simulink model "idq"  (R2021a)
settings: Solver=VariableStepAuto  StartTime=0.0  StopTime=0.2  FixedStep=1/150000  MaxStep=1e-6
undefined symbols (not defined in the file): in, ou
libraries: neural x105, spsMosfetLib x12, simulink x5, pid_lib x3, spsabctodq0Lib x3, spsFirstOrderFilterLib x2, spsPermanentMagnetSynchronousMachineLib x2, spsCurrentMeasurementLib x2, spsDCVoltageSourceLib x2, spsThreePhaseVIMeasurementLib x2, spsabctoAlphaBetaZeroLib x2, spsSVPWMGenerator2LevelLib x1
(part 5 of 7)

== system idq/NARX Neural Network - Closed Loop1/Layer 2/Delays 1 ==
  "p{2}" : Inport  PortDimensions=10  SampleTime=1e-05
      mask Display: e = 0.06;c1 = [120 230 180]/255;c2 = ([120 230 180]+0)/(256+128);c3 = ([120 230 180]+128)/(256+128);patch([0 1 1 0],[0 0 1 1],c1);patch([0 1 1 1-e 1-e 0+e],[0 0 1 1-e 0+e 0+e],c2);patch([0 0 1 1-e 0+e 0+e],[0 1 1 1-e 1-e 0+e],c3);plot([0 1 1 0 0],[0 0 1 1 0]);
  mux : Mux  Inputs=1
      mask Display: e = 0.06;c1 = [120 150 230]/255;c2 = ([120 150 230]+0)/383;c3 = ([120 150 230]+128)/383;patch([0 1 1 0],[0 0 1 1],c1);patch([0 1 1 1-e 1-e 0+e],[0 0 1 1-e 0+e 0+e],c2);patch([0 0 1 1-e 0+e 0+e],[0 1 1 1-e 1-e 0+e],c3);plot([0 1 1 0 0],[0 0 1 1 0]);disp('Mux')
  "pd{2,1}" : Outport
      mask Display: e = 0.06;c1 = [120 230 180]/255;c2 = ([120 230 180]+0)/(256+128);c3 = ([120 230 180]+128)/(256+128);patch([0 1 1 0],[0 0 1 1],c1);patch([0 1 1 1-e 1-e 0+e],[0 0 1 1-e 0+e 0+e],c2);patch([0 0 1 1-e 0+e 0+e],[0 1 1 1-e 1-e 0+e],c3);plot([0 1 1 0 0],[0 0 1 1 0]);
  wires:
  "p{2}"/1 -> mux/1
  mux/1 -> "pd{2,1}"/1

== system idq/NARX Neural Network - Closed Loop1/Layer 2/LW{2,1} ==
  "ad{2,1}" : Inport  PortDimensions=10  SampleTime=1e-05
      mask Display: e = 0.06;c1 = [120 230 180]/255;c2 = ([120 230 180]+0)/(256+128);c3 = ([120 230 180]+128)/(256+128);patch([0 1 1 0],[0 0 1 1],c1);patch([0 1 1 1-e 1-e 0+e],[0 0 1 1-e 0+e 0+e],c2);patch([0 0 1 1-e 0+e 0+e],[0 1 1 1-e 1-e 0+e],c3);plot([0 1 1 0 0],[0 0 1 1 0]);
  "IW{2,1}(1,:)'" : Constant  Value=[0.56153761305586458174587960456847213208675384521484375;0.83032986406449749150482375625870190560817718505859375;1.7572116988873085485778346992447040975093841552734375;-1.22353547781027049978774812188930809497833251953125;0.69692667626243232081861833648872561752796173095703125;1.5315847736811942780832396238110959529876708984375;-1.373036182446984110328003225731663405895233154296875;1.3479512008090404062699008136405609548091888427734375;1.708104159078249306702446119743399322032928466796875;-0.5444366534227558229730448147165589034557342529296875]
      mask Display: e = 0.06;c1 = [120 150 230]/255;c2 = ([120 150 230]+0)/383;c3 = ([120 150 230]+128)/383;patch([0 1 1 0],[0 0 1 1],c1);patch([0 1 1 1-e 1-e 0+e],[0 0 1 1-e 0+e 0+e],c2);patch([0 0 1 1-e 0+e 0+e],[0 1 1 1-e 1-e 0+e],c3);plot([0 1 1 0 0],[0 0 1 1 0]);disp('weights');
  Mux : Mux  Inputs=1
      mask Display: e = 0.06;c1 = [120 150 230]/255;c2 = ([120 150 230]+0)/383;c3 = ([120 150 230]+128)/383;patch([0 1 1 0],[0 0 1 1],c1);patch([0 1 1 1-e 1-e 0+e],[0 0 1 1-e 0+e 0+e],c2);patch([0 0 1 1-e 0+e 0+e],[0 1 1 1-e 1-e 0+e],c3);plot([0 1 1 0 0],[0 0 1 1 0]);disp('Mux');
  dotprod1 : neural/Weight Functions/dotprod
  "lz{2,1}" : Outport
      mask Display: e = 0.06;c1 = [120 230 180]/255;c2 = ([120 230 180]+0)/(256+128);c3 = ([120 230 180]+128)/(256+128);patch([0 1 1 0],[0 0 1 1],c1);patch([0 1 1 1-e 1-e 0+e],[0 0 1 1-e 0+e 0+e],c2);patch([0 0 1 1-e 0+e 0+e],[0 1 1 1-e 1-e 0+e],c3);plot([0 1 1 0 0],[0 0 1 1 0]);
  wires:
  "IW{2,1}(1,:)'"/1 -> dotprod1/1
  "ad{2,1}"/1 -> dotprod1/2
  dotprod1/1 -> Mux/1
  Mux/1 -> "lz{2,1}"/1

== system idq/NARX Neural Network - Closed Loop2/Layer 1/Delays 1 ==
  "p{1}" : Inport  PortDimensions=4  SampleTime=1e-05
      mask Display: e = 0.06;c1 = [120 230 180]/255;c2 = ([120 230 180]+0)/(256+128);c3 = ([120 230 180]+128)/(256+128);patch([0 1 1 0],[0 0 1 1],c1);patch([0 1 1 1-e 1-e 0+e],[0 0 1 1-e 0+e 0+e],c2);patch([0 0 1 1-e 0+e 0+e],[0 1 1 1-e 1-e 0+e],c3);plot([0 1 1 0 0],[0 0 1 1 0]);
  Delay 1 : UnitDelay  InitialCondition=pi_input_1_delayed_1  SampleTime=1e-05
      mask Display: e = 0.06;c1 = [120 150 230]/255;c2 = ([120 150 230]+0)/383;c3 = ([120 150 230]+128)/383;patch([0 1 1 0],[0 0 1 1],c1);patch([0 1 1 1-e 1-e 0+e],[0 0 1 1-e 0+e 0+e],c2);patch([0 0 1 1-e 0+e 0+e],[0 1 1 1-e 1-e 0+e],c3);plot([0 1 1 0 0],[0 0 1 1 0]);disp('D')
  Delay 10 : UnitDelay  InitialCondition=pi_input_1_delayed_10  SampleTime=1e-05
      mask Display: e = 0.06;c1 = [120 150 230]/255;c2 = ([120 150 230]+0)/383;c3 = ([120 150 230]+128)/383;patch([0 1 1 0],[0 0 1 1],c1);patch([0 1 1 1-e 1-e 0+e],[0 0 1 1-e 0+e 0+e],c2);patch([0 0 1 1-e 0+e 0+e],[0 1 1 1-e 1-e 0+e],c3);plot([0 1 1 0 0],[0 0 1 1 0]);disp('D')
  Delay 2 : UnitDelay  InitialCondition=pi_input_1_delayed_2  SampleTime=1e-05
      mask Display: e = 0.06;c1 = [120 150 230]/255;c2 = ([120 150 230]+0)/383;c3 = ([120 150 230]+128)/383;patch([0 1 1 0],[0 0 1 1],c1);patch([0 1 1 1-e 1-e 0+e],[0 0 1 1-e 0+e 0+e],c2);patch([0 0 1 1-e 0+e 0+e],[0 1 1 1-e 1-e 0+e],c3);plot([0 1 1 0 0],[0 0 1 1 0]);disp('D')
  Delay 3 : UnitDelay  InitialCondition=pi_input_1_delayed_3  SampleTime=1e-05
      mask Display: e = 0.06;c1 = [120 150 230]/255;c2 = ([120 150 230]+0)/383;c3 = ([120 150 230]+128)/383;patch([0 1 1 0],[0 0 1 1],c1);patch([0 1 1 1-e 1-e 0+e],[0 0 1 1-e 0+e 0+e],c2);patch([0 0 1 1-e 0+e 0+e],[0 1 1 1-e 1-e 0+e],c3);plot([0 1 1 0 0],[0 0 1 1 0]);disp('D')
  Delay 4 : UnitDelay  InitialCondition=pi_input_1_delayed_4  SampleTime=1e-05
      mask Display: e = 0.06;c1 = [120 150 230]/255;c2 = ([120 150 230]+0)/383;c3 = ([120 150 230]+128)/383;patch([0 1 1 0],[0 0 1 1],c1);patch([0 1 1 1-e 1-e 0+e],[0 0 1 1-e 0+e 0+e],c2);patch([0 0 1 1-e 0+e 0+e],[0 1 1 1-e 1-e 0+e],c3);plot([0 1 1 0 0],[0 0 1 1 0]);disp('D')
  Delay 5 : UnitDelay  InitialCondition=pi_input_1_delayed_5  SampleTime=1e-05
      mask Display: e = 0.06;c1 = [120 150 230]/255;c2 = ([120 150 230]+0)/383;c3 = ([120 150 230]+128)/383;patch([0 1 1 0],[0 0 1 1],c1);patch([0 1 1 1-e 1-e 0+e],[0 0 1 1-e 0+e 0+e],c2);patch([0 0 1 1-e 0+e 0+e],[0 1 1 1-e 1-e 0+e],c3);plot([0 1 1 0 0],[0 0 1 1 0]);disp('D')
  Delay 6 : UnitDelay  InitialCondition=pi_input_1_delayed_6  SampleTime=1e-05
      mask Display: e = 0.06;c1 = [120 150 230]/255;c2 = ([120 150 230]+0)/383;c3 = ([120 150 230]+128)/383;patch([0 1 1 0],[0 0 1 1],c1);patch([0 1 1 1-e 1-e 0+e],[0 0 1 1-e 0+e 0+e],c2);patch([0 0 1 1-e 0+e 0+e],[0 1 1 1-e 1-e 0+e],c3);plot([0 1 1 0 0],[0 0 1 1 0]);disp('D')
  Delay 7 : UnitDelay  InitialCondition=pi_input_1_delayed_7  SampleTime=1e-05
      mask Display: e = 0.06;c1 = [120 150 230]/255;c2 = ([120 150 230]+0)/383;c3 = ([120 150 230]+128)/383;patch([0 1 1 0],[0 0 1 1],c1);patch([0 1 1 1-e 1-e 0+e],[0 0 1 1-e 0+e 0+e],c2);patch([0 0 1 1-e 0+e 0+e],[0 1 1 1-e 1-e 0+e],c3);plot([0 1 1 0 0],[0 0 1 1 0]);disp('D')
  Delay 8 : UnitDelay  InitialCondition=pi_input_1_delayed_8  SampleTime=1e-05
      mask Display: e = 0.06;c1 = [120 150 230]/255;c2 = ([120 150 230]+0)/383;c3 = ([120 150 230]+128)/383;patch([0 1 1 0],[0 0 1 1],c1);patch([0 1 1 1-e 1-e 0+e],[0 0 1 1-e 0+e 0+e],c2);patch([0 0 1 1-e 0+e 0+e],[0 1 1 1-e 1-e 0+e],c3);plot([0 1 1 0 0],[0 0 1 1 0]);disp('D')
  Delay 9 : UnitDelay  InitialCondition=pi_input_1_delayed_9  SampleTime=1e-05
      mask Display: e = 0.06;c1 = [120 150 230]/255;c2 = ([120 150 230]+0)/383;c3 = ([120 150 230]+128)/383;patch([0 1 1 0],[0 0 1 1],c1);patch([0 1 1 1-e 1-e 0+e],[0 0 1 1-e 0+e 0+e],c2);patch([0 0 1 1-e 0+e 0+e],[0 1 1 1-e 1-e 0+e],c3);plot([0 1 1 0 0],[0 0 1 1 0]);disp('D')
  mux : Mux  Inputs=10
      mask Display: e = 0.06;c1 = [120 150 230]/255;c2 = ([120 150 230]+0)/383;c3 = ([120 150 230]+128)/383;patch([0 1 1 0],[0 0 1 1],c1);patch([0 1 1 1-e 1-e 0+e],[0 0 1 1-e 0+e 0+e],c2);patch([0 0 1 1-e 0+e 0+e],[0 1 1 1-e 1-e 0+e],c3);plot([0 1 1 0 0],[0 0 1 1 0]);disp('Mux')
  "pd{1,1}" : Outport
      mask Display: e = 0.06;c1 = [120 230 180]/255;c2 = ([120 230 180]+0)/(256+128);c3 = ([120 230 180]+128)/(256+128);patch([0 1 1 0],[0 0 1 1],c1);patch([0 1 1 1-e 1-e 0+e],[0 0 1 1-e 0+e 0+e],c2);patch([0 0 1 1-e 0+e 0+e],[0 1 1 1-e 1-e 0+e],c3);plot([0 1 1 0 0],[0 0 1 1 0]);
  wires:
  "p{1}"/1 -> Delay 1/1
  Delay 1/1 -> Delay 2/1, mux/1
  Delay 2/1 -> Delay 3/1, mux/2
  Delay 3/1 -> Delay 4/1, mux/3
  Delay 4/1 -> Delay 5/1, mux/4
  Delay 5/1 -> Delay 6/1, mux/5
  Delay 6/1 -> Delay 7/1, mux/6
  Delay 7/1 -> Delay 8/1, mux/7
  Delay 8/1 -> Delay 9/1, mux/8
  Delay 9/1 -> Delay 10/1, mux/9
  Delay 10/1 -> mux/10
  mux/1 -> "pd{1,1}"/1

== system idq/NARX Neural Network - Closed Loop2/Layer 1/Delays 2 ==
  "p{1}" : Inport  PortDimensions=1  SampleTime=1e-05
      mask Display: e = 0.06;c1 = [120 230 180]/255;c2 = ([120 230 180]+0)/(256+128);c3 = ([120 230 180]+128)/(256+128);patch([0 1 1 0],[0 0 1 1],c1);patch([0 1 1 1-e 1-e 0+e],[0 0 1 1-e 0+e 0+e],c2);patch([0 0 1 1-e 0+e 0+e],[0 1 1 1-e 1-e 0+e],c3);plot([0 1 1 0 0],[0 0 1 1 0]);
  Delay 1 : UnitDelay  InitialCondition=ai_layer_2_delayed_1  SampleTime=1e-05
      mask Display: e = 0.06;c1 = [120 150 230]/255;c2 = ([120 150 230]+0)/383;c3 = ([120 150 230]+128)/383;patch([0 1 1 0],[0 0 1 1],c1);patch([0 1 1 1-e 1-e 0+e],[0 0 1 1-e 0+e 0+e],c2);patch([0 0 1 1-e 0+e 0+e],[0 1 1 1-e 1-e 0+e],c3);plot([0 1 1 0 0],[0 0 1 1 0]);disp('D')
  Delay 10 : UnitDelay  InitialCondition=ai_layer_2_delayed_10  SampleTime=1e-05
      mask Display: e = 0.06;c1 = [120 150 230]/255;c2 = ([120 150 230]+0)/383;c3 = ([120 150 230]+128)/383;patch([0 1 1 0],[0 0 1 1],c1);patch([0 1 1 1-e 1-e 0+e],[0 0 1 1-e 0+e 0+e],c2);patch([0 0 1 1-e 0+e 0+e],[0 1 1 1-e 1-e 0+e],c3);plot([0 1 1 0 0],[0 0 1 1 0]);disp('D')
  Delay 2 : UnitDelay  InitialCondition=ai_layer_2_delayed_2  SampleTime=1e-05
      mask Display: e = 0.06;c1 = [120 150 230]/255;c2 = ([120 150 230]+0)/383;c3 = ([120 150 230]+128)/383;patch([0 1 1 0],[0 0 1 1],c1);patch([0 1 1 1-e 1-e 0+e],[0 0 1 1-e 0+e 0+e],c2);patch([0 0 1 1-e 0+e 0+e],[0 1 1 1-e 1-e 0+e],c3);plot([0 1 1 0 0],[0 0 1 1 0]);disp('D')
  Delay 3 : UnitDelay  InitialCondition=ai_layer_2_delayed_3  SampleTime=1e-05
      mask Display: e = 0.06;c1 = [120 150 230]/255;c2 = ([120 150 230]+0)/383;c3 = ([120 150 230]+128)/383;patch([0 1 1 0],[0 0 1 1],c1);patch([0 1 1 1-e 1-e 0+e],[0 0 1 1-e 0+e 0+e],c2);patch([0 0 1 1-e 0+e 0+e],[0 1 1 1-e 1-e 0+e],c3);plot([0 1 1 0 0],[0 0 1 1 0]);disp('D')
  Delay 4 : UnitDelay  InitialCondition=ai_layer_2_delayed_4  SampleTime=1e-05
      mask Display: e = 0.06;c1 = [120 150 230]/255;c2 = ([120 150 230]+0)/383;c3 = ([120 150 230]+128)/383;patch([0 1 1 0],[0 0 1 1],c1);patch([0 1 1 1-e 1-e 0+e],[0 0 1 1-e 0+e 0+e],c2);patch([0 0 1 1-e 0+e 0+e],[0 1 1 1-e 1-e 0+e],c3);plot([0 1 1 0 0],[0 0 1 1 0]);disp('D')
  Delay 5 : UnitDelay  InitialCondition=ai_layer_2_delayed_5  SampleTime=1e-05
      mask Display: e = 0.06;c1 = [120 150 230]/255;c2 = ([120 150 230]+0)/383;c3 = ([120 150 230]+128)/383;patch([0 1 1 0],[0 0 1 1],c1);patch([0 1 1 1-e 1-e 0+e],[0 0 1 1-e 0+e 0+e],c2);patch([0 0 1 1-e 0+e 0+e],[0 1 1 1-e 1-e 0+e],c3);plot([0 1 1 0 0],[0 0 1 1 0]);disp('D')
  Delay 6 : UnitDelay  InitialCondition=ai_layer_2_delayed_6  SampleTime=1e-05
      mask Display: e = 0.06;c1 = [120 150 230]/255;c2 = ([120 150 230]+0)/383;c3 = ([120 150 230]+128)/383;patch([0 1 1 0],[0 0 1 1],c1);patch([0 1 1 1-e 1-e 0+e],[0 0 1 1-e 0+e 0+e],c2);patch([0 0 1 1-e 0+e 0+e],[0 1 1 1-e 1-e 0+e],c3);plot([0 1 1 0 0],[0 0 1 1 0]);disp('D')
  Delay 7 : UnitDelay  InitialCondition=ai_layer_2_delayed_7  SampleTime=1e-05
      mask Display: e = 0.06;c1 = [120 150 230]/255;c2 = ([120 150 230]+0)/383;c3 = ([120 150 230]+128)/383;patch([0 1 1 0],[0 0 1 1],c1);patch([0 1 1 1-e 1-e 0+e],[0 0 1 1-e 0+e 0+e],c2);patch([0 0 1 1-e 0+e 0+e],[0 1 1 1-e 1-e 0+e],c3);plot([0 1 1 0 0],[0 0 1 1 0]);disp('D')
  Delay 8 : UnitDelay  InitialCondition=ai_layer_2_delayed_8  SampleTime=1e-05
      mask Display: e = 0.06;c1 = [120 150 230]/255;c2 = ([120 150 230]+0)/383;c3 = ([120 150 230]+128)/383;patch([0 1 1 0],[0 0 1 1],c1);patch([0 1 1 1-e 1-e 0+e],[0 0 1 1-e 0+e 0+e],c2);patch([0 0 1 1-e 0+e 0+e],[0 1 1 1-e 1-e 0+e],c3);plot([0 1 1 0 0],[0 0 1 1 0]);disp('D')
  Delay 9 : UnitDelay  InitialCondition=ai_layer_2_delayed_9  SampleTime=1e-05
      mask Display: e = 0.06;c1 = [120 150 230]/255;c2 = ([120 150 230]+0)/383;c3 = ([120 150 230]+128)/383;patch([0 1 1 0],[0 0 1 1],c1);patch([0 1 1 1-e 1-e 0+e],[0 0 1 1-e 0+e 0+e],c2);patch([0 0 1 1-e 0+e 0+e],[0 1 1 1-e 1-e 0+e],c3);plot([0 1 1 0 0],[0 0 1 1 0]);disp('D')
  mux : Mux  Inputs=10
      mask Display: e = 0.06;c1 = [120 150 230]/255;c2 = ([120 150 230]+0)/383;c3 = ([120 150 230]+128)/383;patch([0 1 1 0],[0 0 1 1],c1);patch([0 1 1 1-e 1-e 0+e],[0 0 1 1-e 0+e 0+e],c2);patch([0 0 1 1-e 0+e 0+e],[0 1 1 1-e 1-e 0+e],c3);plot([0 1 1 0 0],[0 0 1 1 0]);disp('Mux')
  "pd{1,2}" : Outport
      mask Display: e = 0.06;c1 = [120 230 180]/255;c2 = ([120 230 180]+0)/(256+128);c3 = ([120 230 180]+128)/(256+128);patch([0 1 1 0],[0 0 1 1],c1);patch([0 1 1 1-e 1-e 0+e],[0 0 1 1-e 0+e 0+e],c2);patch([0 0 1 1-e 0+e 0+e],[0 1 1 1-e 1-e 0+e],c3);plot([0 1 1 0 0],[0 0 1 1 0]);
  wires:
  "p{1}"/1 -> Delay 1/1
  Delay 1/1 -> Delay 2/1, mux/1
  Delay 2/1 -> Delay 3/1, mux/2
  Delay 3/1 -> Delay 4/1, mux/3
  Delay 4/1 -> Delay 5/1, mux/4
  Delay 5/1 -> Delay 6/1, mux/5
  Delay 6/1 -> Delay 7/1, mux/6
  Delay 7/1 -> Delay 8/1, mux/7
  Delay 8/1 -> Delay 9/1, mux/8
  Delay 9/1 -> Delay 10/1, mux/9
  Delay 10/1 -> mux/10
  mux/1 -> "pd{1,2}"/1

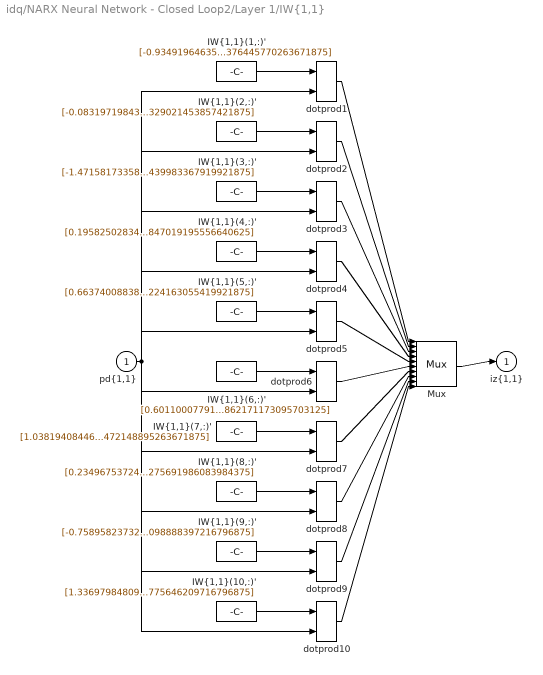
== system idq/NARX Neural Network - Closed Loop2/Layer 1/IW{1,1} ==
  "pd{1,1}" : Inport  PortDimensions=40  SampleTime=1e-05
      mask Display: e = 0.06;c1 = [120 230 180]/255;c2 = ([120 230 180]+0)/(256+128);c3 = ([120 230 180]+128)/(256+128);patch([0 1 1 0],[0 0 1 1],c1);patch([0 1 1 1-e 1-e 0+e],[0 0 1 1-e 0+e 0+e],c2);patch([0 0 1 1-e 0+e 0+e],[0 1 1 1-e 1-e 0+e],c3);plot([0 1 1 0 0],[0 0 1 1 0]);
  "IW{1,1}(1,:)'" : Constant  Value=[-0.93491964635392299509675240187789313495159149169921875;0.5768731944949057055538332861033268272876739501953125;-0.808669545662002775543442112393677234649658203125;1.2749780389204037334138774895109236240386962890625;0.181167627371816630788003976704203523695468902587890625;-0.11293178168770967584322306720423512160778045654296875;-0.60073986928166955845398433666559867560863494873046875;0.96332167376151767168579453937127254903316497802734375;0.661966881594469924721124698407948017120361328125;-0.55526479622883984088588249505846761167049407958984375;-0.413479347827676313453793000007863156497478485107421875;0.6998181089917789865495478807133622467517852783203125;0.356685749586782285813768567095394246280193328857421875;-0.1481556371292291618413372589202481321990489959716796875;-0.2333014868344443770720175734822987578809261322021484375;0.421285328866078001563977295518270693719387054443359375;-0.08821345143658983201095935555713367648422718048095703125;0.33735825315705281202127707729232497513294219970703125;-0.0557309533678579105409056637654430232942104339599609375;0.1184215174993237251754862882080487906932830810546875;0.167721586911953657317297938789124600589275360107421875;-0.33208495241903701611363430856727063655853271484375;0.1215712813527273505886938664843910373747348785400390625;-0.135087992056735439749814986498677171766757965087890625;0.253181771720767223587955641050939448177814483642578125;-0.337459302815608264136670868538203649222850799560546875;0.285806937406632377562942792792455293238162994384765625;-0.37608567364420586454087924721534363925457000732421875;-0.12489555995652874831325362947609391994774341583251953125;0.19080416816666756485432188128470443189144134521484375;0.442239631316194647947526163989095948636531829833984375;-0.645835923498003783294052482233382761478424072265625;0.13085642841257805191190755067509599030017852783203125;0.171765321707068874257373636282864026725292205810546875;0.5737916395563849025762692690477706491947174072265625;-0.90238354543573218169427718748920597136020660400390625;0.11087028890308499307071343764619086869060993194580078125;-0.254177634636488847252877576465834863483905792236328125;0.70197268216156849529596684078569523990154266357421875;-1.129782272419447064493169818888418376445770263671875]
      mask Display: e = 0.06;c1 = [120 150 230]/255;c2 = ([120 150 230]+0)/383;c3 = ([120 150 230]+128)/383;patch([0 1 1 0],[0 0 1 1],c1);patch([0 1 1 1-e 1-e 0+e],[0 0 1 1-e 0+e 0+e],c2);patch([0 0 1 1-e 0+e 0+e],[0 1 1 1-e 1-e 0+e],c3);plot([0 1 1 0 0],[0 0 1 1 0]);disp('Weights');
  "IW{1,1}(10,:)'" : Constant  Value=[1.3369798480945187524326911443495191633701324462890625;0.482692035392721152664563533107866533100605010986328125;-0.46440185193956562414996369625441730022430419921875;-0.28947060915264433145210887232678942382335662841796875;-0.27806839017384243906150231850915588438510894775390625;-0.07654287827070806182749862500713788904249668121337890625;-0.370306883807867304181371537197264842689037322998046875;-0.263686363154703062861017315299250185489654541015625;-0.60337446947651363071685182148939929902553558349609375;-0.145883257794870047074908825379679910838603973388671875;-0.2527720268926625379890538170002400875091552734375;-0.2300477110532727909042449709886568598449230194091796875;-0.054746553261963148973023862708942033350467681884765625;-0.06642024938640662956590432486336794681847095489501953125;-0.1552268451140134952748184105075779370963573455810546875;-0.1719516638105204331399278316894196905195713043212890625;0.26847333459407740630098260226077400147914886474609375;0.0652330438168110815500000398969859816133975982666015625;-0.0694155509714568796919564874770003370940685272216796875;-0.097123765562168340448323533564689569175243377685546875;0.023103300786359082241716578209889121353626251220703125;0.3358079777012061839513989980332553386688232421875;0.0254339133616906278023694909506957628764212131500244140625;-0.0296166842642457961432000956847332417964935302734375;-0.160750306029655842809944488180917687714099884033203125;-0.0411828401246893960330197614894132129848003387451171875;0.1471154645086105716700330958701670169830322265625;0.067279449413947645108891038034926168620586395263671875;0.40692790504593345790596004007966257631778717041015625;0.050840413968451285409155815386839094571769237518310546875;0.2448171162575478454481725520963664166629314422607421875;0.1903632069463795095654035094412392936646938323974609375;0.16899570362654114941136640482000075280666351318359375;0.26196289748042023148855150793679058551788330078125;0.3499685820282956161264564798329956829547882080078125;0.3107483191560700408473394418251700699329376220703125;-0.133099401361700231394280535823781974613666534423828125;-0.042625657158678866009982044715798110701143741607666015625;0.480840149763006596828063266002573072910308837890625;0.455729688087607331947737066002446226775646209716796875]
      mask Display: e = 0.06;c1 = [120 150 230]/255;c2 = ([120 150 230]+0)/383;c3 = ([120 150 230]+128)/383;patch([0 1 1 0],[0 0 1 1],c1);patch([0 1 1 1-e 1-e 0+e],[0 0 1 1-e 0+e 0+e],c2);patch([0 0 1 1-e 0+e 0+e],[0 1 1 1-e 1-e 0+e],c3);plot([0 1 1 0 0],[0 0 1 1 0]);disp('Weights');
  "IW{1,1}(2,:)'" : Constant  Value=[-0.08319719843236932088625934511583182029426097869873046875;-1.194383186937494567558815106167457997798919677734375;-1.3834990018122594879201869844109751284122467041015625;0.0253787429098273654981543501207852386869490146636962890625;-0.05699344337602037235956942140546743758022785186767578125;0.1662986571362562726594802597901434637606143951416015625;-1.1121977649910894658802362755523063242435455322265625;0.0531888285271815419719132478348910808563232421875;0.25383904236635157491974723598104901611804962158203125;0.442519776474258830223362792821717448532581329345703125;-0.84735138876676197039472526739700697362422943115234375;0.059984520283578153521109044277181965298950672149658203125;0.1746526317680719142533263266159337945282459259033203125;0.156708213354486314283775527655961923301219940185546875;-0.55598237448660936532718324087909422814846038818359375;0.06310049190586243528233723054654547013342380523681640625;-0.035454244849806693107296950984164141118526458740234375;-0.2022077526475144770845560060479328967630863189697265625;-0.2298978422451900538447944200015626847743988037109375;0.063403866008216402949670964517281390726566314697265625;0.5124554407111052700685149829951114952564239501953125;0.64457487772015598093133803558885119855403900146484375;0.05983634870600089417091993482245015911757946014404296875;0.0236844005541540260362243230929379933513700962066650390625;-0.021771360218195430491494590796719421632587909698486328125;-0.201292655059645275716917467434541322290897369384765625;0.413102338585970285667059442857862450182437896728515625;-0.0005836268756720529478354553276631122571416199207305908203125;0.270474521102484544154975765195558778941631317138671875;0.057621316576053176194971428003555047325789928436279296875;0.7614393449359708743173769107670523226261138916015625;-0.04165929399175381797615358436814858578145503997802734375;0.1096601608658465398793424583345768041908740997314453125;-0.507756503335163866807988597429357469081878662109375;1.1524614905371792783483897437690757215023040771484375;-0.06760374964590680491038909849521587602794170379638671875;-0.0383894237035154739512421429026289843022823333740234375;0.274172675035019686173853870059247128665447235107421875;1.55013176286031484352179177221842110157012939453125;-0.14902047250095129538038918326492421329021453857421875]
      mask Display: e = 0.06;c1 = [120 150 230]/255;c2 = ([120 150 230]+0)/383;c3 = ([120 150 230]+128)/383;patch([0 1 1 0],[0 0 1 1],c1);patch([0 1 1 1-e 1-e 0+e],[0 0 1 1-e 0+e 0+e],c2);patch([0 0 1 1-e 0+e 0+e],[0 1 1 1-e 1-e 0+e],c3);plot([0 1 1 0 0],[0 0 1 1 0]);disp('Weights');
  "IW{1,1}(3,:)'" : Constant  Value=[-1.47158173358285271348222522647120058536529541015625;0.51193602490896117362950690221623517572879791259765625;-0.144627175018507025949787703211768530309200286865234375;-0.30296090913289541735053944648825563490390777587890625;0.1042062904571169623668680515038431622087955474853515625;-0.2129272579773502649391758723140810616314411163330078125;-0.1029054791512869770908622513161390088498592376708984375;-0.250905250951823088900738412121427245438098907470703125;0.59791582595898906671294525949633680284023284912109375;-0.202153454322915482332945202870178036391735076904296875;-0.08488288559018243584208818219849490560591220855712890625;-0.17619998704942840817011528997682034969329833984375;0.282159260032717573718485937206423841416835784912109375;-0.12070837605131963521376547987529193051159381866455078125;-0.05496612077899332149399924674071371555328369140625;-0.10380002538028076930487486606580205261707305908203125;-0.1254026771991650079929314642868121154606342315673828125;0.12675228429971685528698799316771328449249267578125;-0.012986767998025568193742884659513947553932666778564453125;-0.045090817505936187092885347738047130405902862548828125;-0.1394607879607358824625151783038745634257793426513671875;0.448731616149501355561568516350234858691692352294921875;0.0216616371498709325837950245841057039797306060791015625;0.004625022636832960831743122298576054163277149200439453125;-0.02271964628410023945281892565617454238235950469970703125;-0.346505909292933400589475922970450483262538909912109375;0.0737300929991138997987576431114575825631618499755859375;0.1062770442477673771275448189044254831969738006591796875;-0.053547801662366049935126710579424980096518993377685546875;0.378816082830053024732563926590955816209316253662109375;0.1062060313912706333017155202469439245760440826416015625;0.1783121174015102339271976461532176472246646881103515625;-0.28225371495642381791668640289572067558765411376953125;-0.14447722083072955800986392205231823027133941650390625;0.1620087319721079666123841889202594757080078125;0.27757376681120582428974330468918196856975555419921875;-0.060026201898075115526154377221246249973773956298828125;-0.08062782114587652149140239998814649879932403564453125;0.20233695382172367516204758430831134319305419921875;0.38758942949815355927256632639910094439983367919921875]
      mask Display: e = 0.06;c1 = [120 150 230]/255;c2 = ([120 150 230]+0)/383;c3 = ([120 150 230]+128)/383;patch([0 1 1 0],[0 0 1 1],c1);patch([0 1 1 1-e 1-e 0+e],[0 0 1 1-e 0+e 0+e],c2);patch([0 0 1 1-e 0+e 0+e],[0 1 1 1-e 1-e 0+e],c3);plot([0 1 1 0 0],[0 0 1 1 0]);disp('Weights');
  "IW{1,1}(4,:)'" : Constant  Value=[0.195825028345290752529450628571794368326663970947265625;0.03323717273785516124195993370449286885559558868408203125;1.1422422697764573751300076764891855418682098388671875;-0.1251177032267672128984514756666612811386585235595703125;0.026042306451075754314405941158838686533272266387939453125;0.20398108894994171347292422069585882127285003662109375;0.8807879650031302798396382058854214847087860107421875;-0.132869743338932588816447832869016565382480621337890625;-0.42699371483653358883003647861187346279621124267578125;-0.250251076445925868529940316875581629574298858642578125;0.653748025909990371218327709357254207134246826171875;-0.12147526277643506953385355018326663412153720855712890625;-0.2301580825175155997630582760393735952675342559814453125;0.09072399579929842083902968852271442301571369171142578125;0.409156347397278630229067175605450756847858428955078125;-0.11335276852233509836676006443667574785649776458740234375;0.198524007816302139328712428323342464864253997802734375;0.0237154143093160039990063836512490524910390377044677734375;0.147184552281201364021256949854432605206966400146484375;-0.0812383567752139323925320013586315326392650604248046875;-0.169076260911582731960578485086443834006786346435546875;-0.319543377138391093694735900498926639556884765625;-0.0880963755902458844904145962573238648474216461181640625;-0.03340735323878639417838343206312856636941432952880859375;-0.219808888403599966832047130083083175122737884521484375;0.04215532061683358033832291766884736716747283935546875;-0.33108516405003529659012428965070284903049468994140625;0.00441130039067110131523197225078547489829361438751220703125;-0.2429537497043617599867815215475275181233882904052734375;0.1434244353711615904689580247577396221458911895751953125;-0.57669099223135111831339827404008246958255767822265625;0.04563014775692254831884753230042406357824802398681640625;0.242179973511298773924949045976973138749599456787109375;-0.22415938686366165821794993462390266358852386474609375;-0.836849420385224362917142570950090885162353515625;0.127234272597659181514018200687132775783538818359375;-0.265707414469025848813288348537753336131572723388671875;-0.0223291173543794518874250343287712894380092620849609375;-1.08250534820964361415462917648255825042724609375;0.19539946661073914757622560500749386847019195556640625]
      mask Display: e = 0.06;c1 = [120 150 230]/255;c2 = ([120 150 230]+0)/383;c3 = ([120 150 230]+128)/383;patch([0 1 1 0],[0 0 1 1],c1);patch([0 1 1 1-e 1-e 0+e],[0 0 1 1-e 0+e 0+e],c2);patch([0 0 1 1-e 0+e 0+e],[0 1 1 1-e 1-e 0+e],c3);plot([0 1 1 0 0],[0 0 1 1 0]);disp('Weights');
  "IW{1,1}(5,:)'" : Constant  Value=[0.66374008838757470041258557102992199361324310302734375;1.395565340304592449882647997583262622356414794921875;1.1490574756784519561136903575970791280269622802734375;0.74928721674299547661490805694484151899814605712890625;-0.167338961193904511848273841678746975958347320556640625;-0.294686046563356229821550869019120000302791595458984375;0.89319632496970269297520417239866219460964202880859375;0.6069016943724732104925578823895193636417388916015625;-0.43913901115988529522127237214590422809123992919921875;-0.7326616801190783956343466343241743743419647216796875;0.66674431035242298637655267157242633402347564697265625;0.4708606365220495693080238197580911219120025634765625;-0.10617032880841180408904023124705418013036251068115234375;-0.49972453022129592614675175354932434856891632080078125;0.421981277652361652652501788907102309167385101318359375;0.32308985446238003280683415141538716852664947509765625;0.347846746318644595152846932251122780144214630126953125;0.2225450031572223930087517373976879753172397613525390625;0.13876207076321389610740197895211167633533477783203125;0.141231079174007290166770189898670651018619537353515625;-0.486316727339711596389548731167451478540897369384765625;-0.31561748136346279292041572261950932443141937255859375;-0.08960745953222971904583715740955085493624210357666015625;-0.043261826740486460096679621756265987642109394073486328125;-0.1795106347094850007817257164788316003978252410888671875;-0.3347977017957901590961000692914240062236785888671875;-0.328763216772518518382639740593731403350830078125;-0.226575286696659661256347817470668815076351165771484375;0.1570139353533814563501636030196095816791057586669921875;0.1832039537719976907137464650077163241803646087646484375;-0.59448634625258056640717541085905395448207855224609375;-0.43490652168715981940039227993111126124858856201171875;0.1523770395640471064790943955813418142497539520263671875;0.245248992807236998459075039136223495006561279296875;-0.8567409577658917640974323148839175701141357421875;-0.65259707383066090091716660026577301323413848876953125;-0.159310173544315258897796638848376460373401641845703125;-0.31548239240320352649860069504939019680023193359375;-1.0812774159983657984440696964156813919544219970703125;-0.85730173327215630774134069724823348224163055419921875]
      mask Display: e = 0.06;c1 = [120 150 230]/255;c2 = ([120 150 230]+0)/383;c3 = ([120 150 230]+128)/383;patch([0 1 1 0],[0 0 1 1],c1);patch([0 1 1 1-e 1-e 0+e],[0 0 1 1-e 0+e 0+e],c2);patch([0 0 1 1-e 0+e 0+e],[0 1 1 1-e 1-e 0+e],c3);plot([0 1 1 0 0],[0 0 1 1 0]);disp('Weights');
  "IW{1,1}(6,:)'" : Constant  Value=[0.601100077918623743045145602081902325153350830078125;1.6348028861509165121645992257981561124324798583984375;0.39907146896757605958327985717914998531341552734375;-1.0875335124255236518564515790785662829875946044921875;-0.1713856334569804629186506872429163195192813873291015625;-0.3431898993502533468102910774177871644496917724609375;0.30419634141477625011162899681949056684970855712890625;-0.82649108062064780000355312949977815151214599609375;-0.29012445512841311678897682213573716580867767333984375;-0.771433339795148498296839534305036067962646484375;0.23464953170495250756033556172042153775691986083984375;-0.55210194948628987798855405344511382281780242919921875;-0.1811800752743187026272408957083825953304767608642578125;-0.046390013259686550817217920439361478202044963836669921875;0.1461037748507073852355375720435404218733310699462890625;-0.31678231020277924923078671781695447862148284912109375;-0.034112533324353655483918146273936145007610321044921875;0.28925173076399801619373874927987344563007354736328125;0.0473256066241039830000403298981836996972560882568359375;-0.1011515195387369392410192858733353205025196075439453125;-0.1478375590103229442195953424743493087589740753173828125;0.440512282584025915976866372147924266755580902099609375;-0.04665042900509684675736110648358589969575405120849609375;0.09953303567979628063699948370413039810955524444580078125;-0.09657792128406077203361945748838479630649089813232421875;-0.25476319129673907770694540886324830353260040283203125;-0.11725750095708893649959492222478729672729969024658203125;0.333228913226925993473770404307288117706775665283203125;0.04717171828468114114230047562159597873687744140625;0.490868316683557404100923804435296915471553802490234375;-0.209150212539155944124757979807327501475811004638671875;0.529596749138641964549378826632164418697357177734375;-8.9550877950498632140696741998908692039549350738525390625e-05;0.261939163832486887617534421224263496696949005126953125;-0.283414961804948128953896002713008783757686614990234375;0.73495334337888584830267291181371547281742095947265625;-0.0994682167571795117222421822589240036904811859130859375;-0.189395485566832111334889532372471876442432403564453125;-0.32772915193615492768230978981591761112213134765625;0.9594566303287532793575564937782473862171173095703125]
      mask Display: e = 0.06;c1 = [120 150 230]/255;c2 = ([120 150 230]+0)/383;c3 = ([120 150 230]+128)/383;patch([0 1 1 0],[0 0 1 1],c1);patch([0 1 1 1-e 1-e 0+e],[0 0 1 1-e 0+e 0+e],c2);patch([0 0 1 1-e 0+e 0+e],[0 1 1 1-e 1-e 0+e],c3);plot([0 1 1 0 0],[0 0 1 1 0]);disp('Weights');
  "IW{1,1}(7,:)'" : Constant  Value=[1.0381940844642827403987439538468606770038604736328125;-0.145515017117523459688754883245564997196197509765625;0.108477901161546486097364550005295313894748687744140625;-0.60516176759280038144339641803526319563388824462890625;-0.3892498657522340810288596912869252264499664306640625;-0.2055866513737691081420422278824844397604465484619140625;0.09585907034366709933426164980119210667908191680908203125;-0.496136068695633591918436877676867879927158355712890625;-0.302479525743452104524777723781880922615528106689453125;0.445645153340425703714089422646793536841869354248046875;0.06127711528414007957632492207267205230891704559326171875;-0.408090481284177963861026228187256492674350738525390625;-0.203684871032761283249357120439526624977588653564453125;-0.1601468665782785072426719352733925916254520416259765625;0.0401954789074373819435237464858801104128360748291015625;-0.277128772005242274278913328089402057230472564697265625;0.1166618351515140428187322640951606445014476776123046875;-0.1156738931758617139333722434457740746438503265380859375;0.00411272176279790270536640406362494104541838169097900390625;-0.1289177250203636104775029025404364801943302154541015625;-0.387827676771339557859619162627495825290679931640625;0.34388919240182802550265250829397700726985931396484375;-0.0203422616890869580041911746093319379724562168121337890625;-0.00882045119323031541480606421146148932166397571563720703125;-0.07866850738171375645446659063964034430682659149169921875;0.05093454098443843391930130337641458027064800262451171875;-0.0499903892377522307555182123905979096889495849609375;0.1439560109670901255629615889120032079517841339111328125;0.290769735176010402089019635241129435598850250244140625;0.0276199189578246462328792176776914857327938079833984375;-0.0961359023445205185254280877416022121906280517578125;0.317279533480216147101060641944059170782566070556640625;0.0012857170992351119043206608694163151085376739501953125;0.0181113181443570796236297582026963937096297740936279296875;-0.1305028229391014260585279771476052701473236083984375;0.491678280028801928391857245514984242618083953857421875;-0.171037030276247226101560272581991739571094512939453125;0.0942413697691943663681257703501614741981029510498046875;-0.162311469350189085947278044841368682682514190673828125;0.6671410707774725334928689335356466472148895263671875]
      mask Display: e = 0.06;c1 = [120 150 230]/255;c2 = ([120 150 230]+0)/383;c3 = ([120 150 230]+128)/383;patch([0 1 1 0],[0 0 1 1],c1);patch([0 1 1 1-e 1-e 0+e],[0 0 1 1-e 0+e 0+e],c2);patch([0 0 1 1-e 0+e 0+e],[0 1 1 1-e 1-e 0+e],c3);plot([0 1 1 0 0],[0 0 1 1 0]);disp('Weights');
  "IW{1,1}(8,:)'" : Constant  Value=[0.2349675372411852425358347318251617252826690673828125;0.4128164243049514681160871987231075763702392578125;-0.486118905922806099351163311439449898898601531982421875;0.1430931249202506416740021677469485439360141754150390625;-0.325354781542076365585813846337259747087955474853515625;-0.1119778984232733531900549905913067050278186798095703125;-0.373340955862519641161867411938146688044071197509765625;0.11557373184287637879474885949093732051551342010498046875;0.18774291010160248927007842212333343923091888427734375;0.0109818993608117587701400452715461142361164093017578125;-0.283958333855399647216444236619281582534313201904296875;0.090526580603283779424828026094473898410797119140625;-0.03383985902405116374946913992971531115472316741943359375;-0.18642315338833037596799613311304710805416107177734375;-0.1753761362418959357523107200904632918536663055419921875;0.0646690535685037481972159412180189974606037139892578125;-0.057044731422148019228668403002302511595189571380615234375;0.259055236021593249251537827149149961769580841064453125;-0.07463877129435132762313998000536230392754077911376953125;0.0101685269016420047616389155109573039226233959197998046875;0.1943321810553335360349791471890057437121868133544921875;-0.26000303363224064323588891056715510785579681396484375;0.032253756660963757429971821011349675245583057403564453125;-0.015600486434286763015588661573929130099713802337646484375;0.0776867671826327044204418825756874866783618927001953125;0.1386078009799963373094300322918570600450038909912109375;0.136991337684286895726160082631395198404788970947265625;-0.06904070311945394167185696687738527543842792510986328125;-0.124584033504338387299270607400103472173213958740234375;-0.11147277527595149393402351734039257280528545379638671875;0.262260094674134192072045834720483981072902679443359375;-0.1196900331105906489792545244199573062360286712646484375;0.2083335416912474313821945770541788078844547271728515625;0.48822747336876870516420012791058979928493499755859375;0.359743685401678003898950919392518699169158935546875;-0.1959675280863937552044973244846914894878864288330078125;-0.10048141629017139087043375411667511798441410064697265625;-0.2248875061175976963756539817040902562439441680908203125;0.497221423016258212701501406627357937395572662353515625;-0.2486908957496215266669281618305831216275691986083984375]
      mask Display: e = 0.06;c1 = [120 150 230]/255;c2 = ([120 150 230]+0)/383;c3 = ([120 150 230]+128)/383;patch([0 1 1 0],[0 0 1 1],c1);patch([0 1 1 1-e 1-e 0+e],[0 0 1 1-e 0+e 0+e],c2);patch([0 0 1 1-e 0+e 0+e],[0 1 1 1-e 1-e 0+e],c3);plot([0 1 1 0 0],[0 0 1 1 0]);disp('Weights');
  "IW{1,1}(9,:)'" : Constant  Value=[-0.75895823732300582431520297177485190331935882568359375;-0.100409152538610213500902546002180315554141998291015625;-0.054249198935480628935845714977403986267745494842529296875;0.03665591781840003837711350342942751012742519378662109375;0.13938949451906690324420878823730163276195526123046875;0.12473897230672659208750019388389773666858673095703125;-0.052967310352746481416641444184278952889144420623779296875;0.04956175642803915815104431885629310272634029388427734375;0.19348408571919140097605804839986376464366912841796875;0.1650096406465207110603188311870326288044452667236328125;-0.05281502391079216651714745012213825248181819915771484375;0.05344697692106596675909457871966878883540630340576171875;0.30645873210301688427392718949704430997371673583984375;-0.02141018597143051760411935902084223926067352294921875;-0.050106590295544262136928637119126506149768829345703125;0.061222168231805117188937259697922854684293270111083984375;0.1991326386390174507656780633624293841421604156494140625;0.244114778014751399037862711338675580918788909912109375;-0.04815438234738829426095918506689486093819141387939453125;0.044249952669205609712133053790239500813186168670654296875;-0.52946456604212688290544974734075367450714111328125;-0.60817951768132305634395606830366887152194976806640625;0.01328708829746189264142675057200904120691120624542236328125;0.0441493579093733823359713142053806222975254058837890625;0.151845388316959539753980834575486369431018829345703125;0.128405127431829690909381724850391037762165069580078125;0.0249302849033115891952405718257068656384944915771484375;0.017921732975081428040908804177888669073581695556640625;-0.09747667535201720578896811275626532733440399169921875;0.11404510143885608630665018381478148512542247772216796875;0.05104641402608499356485793896354152821004390716552734375;-0.0212531933600250029503531123964421567507088184356689453125;0.03711230700920543912335602954044588841497898101806640625;0.22617236406578589136273649273789487779140472412109375;0.07225801560207316398543042623714427463710308074951171875;-0.0678705871736762500479045456813764758408069610595703125;-0.0703815385852742669836601407951093278825283050537109375;-0.218311240658921656976332315025501884520053863525390625;0.1178367705339280757659281562155229039490222930908203125;-0.1016146142867888346739135840834933333098888397216796875]
      mask Display: e = 0.06;c1 = [120 150 230]/255;c2 = ([120 150 230]+0)/383;c3 = ([120 150 230]+128)/383;patch([0 1 1 0],[0 0 1 1],c1);patch([0 1 1 1-e 1-e 0+e],[0 0 1 1-e 0+e 0+e],c2);patch([0 0 1 1-e 0+e 0+e],[0 1 1 1-e 1-e 0+e],c3);plot([0 1 1 0 0],[0 0 1 1 0]);disp('Weights');
  Mux : Mux  Inputs=10
      mask Display: e = 0.06;c1 = [120 150 230]/255;c2 = ([120 150 230]+0)/383;c3 = ([120 150 230]+128)/383;patch([0 1 1 0],[0 0 1 1],c1);patch([0 1 1 1-e 1-e 0+e],[0 0 1 1-e 0+e 0+e],c2);patch([0 0 1 1-e 0+e 0+e],[0 1 1 1-e 1-e 0+e],c3);plot([0 1 1 0 0],[0 0 1 1 0]);disp('Mux');
  dotprod{1..10} (10 alike) : neural/Weight Functions/dotprod
  "iz{1,1}" : Outport
      mask Display: e = 0.06;c1 = [120 230 180]/255;c2 = ([120 230 180]+0)/(256+128);c3 = ([120 230 180]+128)/(256+128);patch([0 1 1 0],[0 0 1 1],c1);patch([0 1 1 1-e 1-e 0+e],[0 0 1 1-e 0+e 0+e],c2);patch([0 0 1 1-e 0+e 0+e],[0 1 1 1-e 1-e 0+e],c3);plot([0 1 1 0 0],[0 0 1 1 0]);
  wires:
  "IW{1,1}(1,:)'"/1 -> dotprod1/1
  "pd{1,1}"/1 -> dotprod1/2, dotprod2/2, dotprod3/2, dotprod4/2, dotprod5/2, dotprod6/2, dotprod7/2, dotprod8/2, dotprod9/2, dotprod10/2
  dotprod1/1 -> Mux/1
  "IW{1,1}(2,:)'"/1 -> dotprod2/1
  dotprod2/1 -> Mux/2
  "IW{1,1}(3,:)'"/1 -> dotprod3/1
  dotprod3/1 -> Mux/3
  "IW{1,1}(4,:)'"/1 -> dotprod4/1
  dotprod4/1 -> Mux/4
  "IW{1,1}(5,:)'"/1 -> dotprod5/1
  dotprod5/1 -> Mux/5
  "IW{1,1}(6,:)'"/1 -> dotprod6/1
  dotprod6/1 -> Mux/6
  "IW{1,1}(7,:)'"/1 -> dotprod7/1
  dotprod7/1 -> Mux/7
  "IW{1,1}(8,:)'"/1 -> dotprod8/1
  dotprod8/1 -> Mux/8
  "IW{1,1}(9,:)'"/1 -> dotprod9/1
  dotprod9/1 -> Mux/9
  "IW{1,1}(10,:)'"/1 -> dotprod10/1
  dotprod10/1 -> Mux/10
  Mux/1 -> "iz{1,1}"/1
